simulink model "SimpleScenarioAndSensorModel3DSimulation"  (R2020a)
settings: Solver=FixedStepAuto  StartTime=0.0  StopTime=30.0  RelTol=1e-3
undefined symbols (not defined in the file or in its folder): f
libraries: etargetslib x3, sim3dautolib x3, instrumentlib x3, sim3dlib x1, autolibshared x1
settings Model: EnablePacing=on  Creator=The MathWorks, Inc.  LastModifiedBy=javot
settings DebuggingCC: SymbolicDimsDataTypeCodeGenerationDiagnostic=none

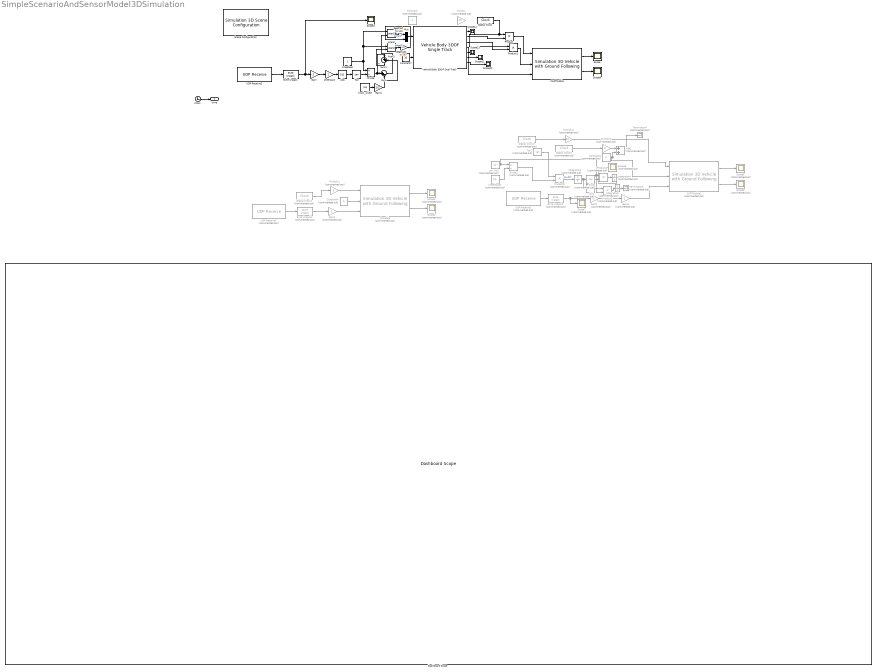
== system SimpleScenarioAndSensorModel3DSimulation ==
  Abs : Abs
  Add1 : Sum  Commented=on
  Atan1 : Trigonometry  Operator=atan2
  Atan2 : Trigonometry  Operator=atan2
  Byte Unpack : etargetslib/Byte Unpack  dimensions={[1]}  datatypes={'double'}  byteAlign=1
  Byte Unpack1 : etargetslib/Byte Unpack  Commented=on  dimensions={[1]}  datatypes={'double'}  byteAlign=1
  Byte Unpack2 : etargetslib/Byte Unpack  Commented=on  dimensions={[1]}  datatypes={'double'}  byteAlign=1
  CAPTMobile : sim3dautolib/Simulation 3D Vehicle with Ground Following  Priority=-1  PassVehMesh=Sport utility vehicle  VehColor=Blue  InitialPos=[10, 0, 0]  InitialRot=[0, 0, 90]  ActorName=CAPTMobile  SampleTime=-1  ActorType=SimulinkVehicle  ID=C  aMode=3  ActorTag=CAPTMobile  CoordinateScheme=ISO  TransformOutportEnabled=on
      settings: SourceProductBaseCode=DR,VE
  CAPTMobile1 : sim3dautolib/Simulation 3D Vehicle with Ground Following  Priority=-1  Commented=on  PassVehMesh=Sport utility vehicle  VehColor=Blue  InitialPos=[10, 0, 0]  InitialRot=[0, 0, 90]  ActorName=SimulinkVehicle1  SampleTime=-1  ActorType=SimulinkVehicle  ID=1  aMode=3  ActorTag=SimulinkVehicle1  CoordinateScheme=ISO  TransformOutportEnabled=on
      settings: SourceProductBaseCode=DR,VE
  Clock : Clock
  Constant : Constant  Commented=on  Value=0
  Constant3 : Constant  Commented=on  Value=0
  Constant4 : Constant  Commented=on  Value=0
  Constant7 : Constant  Value=10
  Cos1 : Trigonometry  Commented=on  Operator=cos
  Dashboard Scope : DashboardScope
  Digital Clock : DigitalClock  SampleTime=0.01
  Digital Clock1 : DigitalClock  Commented=on  SampleTime=0.01
  Digital Clock2 : DigitalClock  Commented=on  SampleTime=0.01
  Digital Clock3 : DigitalClock  Commented=on  SampleTime=0.01
  Divide : Product  Inputs=*/
  Divide1 : Product  Commented=on  Inputs=*/
  Gain : Gain  Gain=-1
  Gain1 : Gain  Gain=1/2
  Gain2 : Gain  Commented=on  Gain=-1
  Gain3 : Gain  Commented=on
  Gain4 : Gain  Commented=on  Gain=-1
  Integrator3 : Integrator  Commented=on
  Integrator4 : Integrator  Commented=on
  Integrator5 : Integrator  Commented=on
  Mozabile : sim3dautolib/Simulation 3D Vehicle with Ground Following  Priority=-1  Commented=on  PassVehMesh=Sport utility vehicle  VehColor=Blue  InitialPos=[20, 10, 0]  InitialRot=[0, 0, 90]  ActorName=SimulinkVehicle2  SampleTime=-1  ActorType=SimulinkVehicle  ID=2  aMode=3  ActorTag=SimulinkVehicle2  CoordinateScheme=ISO  TransformOutportEnabled=on
      settings: SourceProductBaseCode=DR,VE
  Multiply : Gain  Commented=on  Gain=20
  Multiply1 : Gain  Commented=on  Gain=5
  Multiply2 : Gain  Commented=on  Gain=10
  Multiply3 : Gain  Commented=on  Gain=0
  Mux : Mux  Inputs=2
  Product : Product
  Product1 : Product
  Product3 : Product  Commented=on
  Product4 : Product  Commented=on
  Product5 : Product  Commented=on
  Scene Configuration : sim3dlib/Simulation 3D Scene Configuration  Priority=0  ProjectFormat=Default Scenes  SceneDesc=Straight road  ProjectName=VehicleSimulation.exe  ScenePath=/Game/Maps/HwStrght  vehTagList={'CAPTMobile';'Scene Origin';'SimulinkVehicle1';'SimulinkVehicle2'}  vehTag=CAPTMobile  OpVisEn=off  Ts=1/100  EnableWindow=on  sensorTag=MainCamera2  sensorId=2  sensorName=MainCamera2  mountLoc=Origin  offsetFlag=off  tmountOffset=[0, 0, 0]  rmountOffset=[0, 0, 0]  HorizontalResolution=1280  VerticalResolution=720  HorizontalFOV=60  mountPoint=[0 0 0]  mountOrientation=[0 0 0]  aMode=3  ID=2
      settings: SourceProductBaseCode=DR,VE
  Scope{,1,5,11..14} (7 alike) : Scope
  Scope{2..3,6..9} (6 alike) : Scope  Commented=on
  Sin1 : Trigonometry  Commented=on
  Sum : Sum  Inputs=|+-
  Sum1 : Sum  Inputs=|++
  Tan : Trigonometry  Operator=tan
  Tan1 : Trigonometry  Commented=on  Operator=tan
  Terminator3 : Terminator  Commented=on
  Terminator4 : Terminator  Commented=on
  UDP Receive1 : instrumentlib/UDP Receive  Commented=on  Host=localhost  Port=55001  LocalPort=55001  EnablePortSharing=off  GetLatestData=on  DataSize=8  DataType=uint8  ASCIIFormatting=%f,  Terminator=LF  ByteOrder=BigEndian  EnableBlockingMode=on  Timeout=10  SampleTime=0.01  LocalAddress=134.105.60.99
  UDP Receive2 : instrumentlib/UDP Receive  Host=localhost  Port=5006  LocalPort=5006  EnablePortSharing=off  GetLatestData=on  DataSize=8  DataType=uint8  ASCIIFormatting=%f,  Terminator=LF  ByteOrder=LittleEndian  EnableBlockingMode=on  Timeout=10  SampleTime=0.01  LocalAddress=127.0.0.1
  UDP Receive3 : instrumentlib/UDP Receive  Commented=on  Host=localhost  Port=55001  LocalPort=55001  EnablePortSharing=off  GetLatestData=on  DataSize=8  DataType=uint8  ASCIIFormatting=%f,  Terminator=LF  ByteOrder=BigEndian  EnableBlockingMode=on  Timeout=10  SampleTime=0.01  LocalAddress=134.105.60.99
  Vehicle Body 3DOF Dual Track : autolibshared/Vehicle Body 3DOF Single Track  trackMode=Dual  inputMode=External longitudinal velocity  frontSteerMode=on  rearSteerMode=off  windMode=off  muMode=off  extFMode=off  extMMode=off  extXo=off  extpsio=off  extxdoto=off  extro=off  extYo=off  extTamb=off  extydoto=off  aMode=2  NF=2  NR=2  m=2000  a=1.4  b=1.6  h=0.35  X_o=0  xdot_o=0  CalphaMode=off  sigmaMode=on  d=0  w=[1.4,1.4]  Cy_f=12e3  Cy_r=11e3  sigma_f=.1  sigma_r=.1  alpha_f_brk=[-.1 .1]  Cy_f_data=[-9e3 9e3]  alpha_r_brk=[-.1 .1]  Cy_r_data=[-9e3 9e3]  Y_o=0  ydot_o=0  Izz=4000  psi_o=0  r_o=0  Af=2  Cd=.3  Cl=.1  Cpm=.1  beta_w=[0:0.01:0.3]  Cs=[0:0.03:0.9]  Cym=[0:0.01:0.3]  Pabs=101325  Tair=273  g=9.81  mu=1  xdot_tol=.01  Fznom=5000  Fxtire_sat=7e4  Fytire_sat=7e4  longOff=0  latOff=0  vertOff=0  wrapAng=off
      settings: SourceProductBaseCode=PW,MT,VE,VP
  car_vel1 : Constant  Commented=on  Value=10
  deg2rad : Gain  Gain=pi/180
  deg2rad1 : Gain  Gain=pi/180
  steer2act : Gain
  track_width : Constant  Value=0.8
  wheelbae : Constant
  wheelbase1 : Constant  Commented=on  Value=0.1
  time : Outport
  wires:
  CAPTMobile/1 -> Scope/1
  CAPTMobile/2 -> Scope5/1
  Clock/1 -> time/1
  Add1/1 -> Terminator4/1
  Product5/1 -> Integrator5/1
  Gain3/1 -> CAPTMobile1/3
  wheelbase1/1 -> Divide1/2
  Integrator5/1 -> Terminator3/1
  Product3/1 -> Integrator3/1  "psi_dot"
  Integrator3/1 -> Sin1/1, Cos1/1
  Sin1/1 -> Product5/1
  Digital Clock3/1 -> Multiply3/1
  Digital Clock2/1 -> Multiply2/1
  Product4/1 -> Integrator4/1
  Multiply2/1 -> CAPTMobile1/1
  Constant3/1 -> Add1/2, CAPTMobile1/2
  Cos1/1 -> Product4/2
  Multiply3/1 -> Add1/1
  Tan1/1 -> Product3/1
  CAPTMobile1/1 -> Scope6/1
  UDP Receive3/1 -> Byte Unpack1/1
  car_vel1/1 -> Product5/2, Product4/1, Divide1/1
  CAPTMobile1/2 -> Scope9/1
  Integrator4/1 -> Scope8/1
  Divide1/1 -> Product3/2
  Gain2/1 -> Gain3/1
  Byte Unpack1/1 -> Scope7/1, Gain2/1
  Mozabile/2 -> Scope2/1
  Mozabile/1 -> Scope3/1
  Byte Unpack2/1 -> Gain4/1
  Gain4/1 -> Mozabile/3
  Constant4/1 -> Mozabile/2
  Multiply1/1 -> Mozabile/1
  Digital Clock1/1 -> Multiply1/1
  UDP Receive1/1 -> Byte Unpack2/1
  UDP Receive2/1 -> Byte Unpack/1
  Byte Unpack/1 -> Gain/1, Scope1/1
  Vehicle Body 3DOF Dual Track/2 -> Product/2
  Product/1 -> CAPTMobile/1
  Product1/1 -> CAPTMobile/2
  Digital Clock/1 -> Product1/1, Product/1
  Vehicle Body 3DOF Dual Track/3 -> Product1/2
  Vehicle Body 3DOF Dual Track/4 -> CAPTMobile/3
  Vehicle Body 3DOF Dual Track/5 -> Scope13/1
  Vehicle Body 3DOF Dual Track/6 -> Scope11/1
  Vehicle Body 3DOF Dual Track/7 -> Scope12/1
  Constant7/1 -> Vehicle Body 3DOF Dual Track/2
  Vehicle Body 3DOF Dual Track/1 -> Scope14/1
  Gain/1 -> steer2act/1
  steer2act/1 -> Abs/1
  Abs/1 -> Tan/1
  Tan/1 -> Divide/2
  wheelbae/1 -> Atan1/1, Atan2/1, Divide/1
  track_width/1 -> Gain1/1
  Divide/1 -> Sum1/1, Sum/1  "R"
  Gain1/1 -> Sum1/2, Sum/2
  Sum/1 -> Atan2/2
  Sum1/1 -> Atan1/2
  Mux/1 -> Vehicle Body 3DOF Dual Track/1
  Atan2/1 -> deg2rad/1  "deltaFL"
  deg2rad/1 -> Mux/1
  Atan1/1 -> deg2rad1/1  "deltaFR"
  deg2rad1/1 -> Mux/2
